simulink model "dynamiczny_dyskretny_for_print"  (R2020a)
settings: Solver=VariableStepAuto  StartTime=0.0  StopTime=10.0  RelTol=1e-3
values from neighbouring files (symbols this model uses):
  a1 = 0.56    [init_values.m]
  a2 = -0.8    [init_values.m]
  a3 = -0.25    [init_values.m]
  a4 = 0.2    [init_values.m]
  K = 4    [init_values.m]
  T = 1    [test.m]    (also in zad1_10.m; zad1_3.m = 0.1; zad1_9.m)
  T1 = 4    [init_values.m]
  T2 = 10    [init_values.m]
settings Model: Creator=jakub  LastModifiedBy=jakub

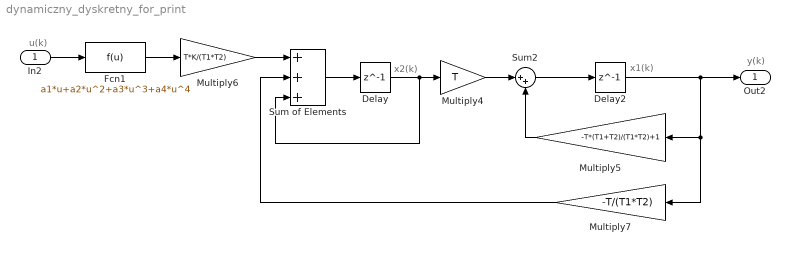
== system dynamiczny_dyskretny_for_print ==
  note: y(k)
  note: u(k)
  note: x1(k)
  note: x2(k)
  In2 : Inport
  Delay : Delay  DelayLength=1  InitialCondition=0
  Delay2 : Delay  DelayLength=1  InitialCondition=0
  Fcn1 : Fcn  Expr=a1*u+a2*u^2+a3*u^3+a4*u^4
  Multiply4 : Gain  Gain=T
  Multiply5 : Gain  Gain=-T*(T1+T2)/(T1*T2)+1
  Multiply6 : Gain  Gain=T*K/(T1*T2)
  Multiply7 : Gain  Gain=-T/(T1*T2)
  Sum of Elements : Sum  Inputs=+++
  Sum2 : Sum  Inputs=|++
  Out2 : Outport
  wires:
  Sum2/1 -> Delay2/1
  Delay/1 -> Sum of Elements/3, Multiply4/1
  Multiply4/1 -> Sum2/1
  Delay2/1 -> Out2/1, Multiply5/1, Multiply7/1
  Multiply5/1 -> Sum2/2
  In2/1 -> Fcn1/1
  Fcn1/1 -> Multiply6/1
  Multiply6/1 -> Sum of Elements/1
  Multiply7/1 -> Sum of Elements/2
  Sum of Elements/1 -> Delay/1
